simulink model "roll_loop"  (Simulink 9.1)
settings: Solver=VariableStepAuto  StartTime=0.0  StopTime=20  RelTol=1e-3
InitFcn:
  | param_chap6
undefined symbols (not defined in the file): G
libraries: simulink x1, cstblocks x1
settings Model: Creator=leonardopedroso  LastModifiedBy=João Pinto
settings DataIOCC: SaveFormat=Dataset
settings OptimizationCC: LifeSpan=auto
settings DebuggingCC: UnderspecifiedInitializationDetection=Simplified  MergeDetectMultiDrivingBlocksExec=error  SFUnexpectedBacktrackingDiag=error  SFNoUnconditionalDefaultTransitionDiag=error  SFExecutionAtInitializationDiag=warning
settings HardwareCC: ProdBitPerPointer=64  ProdBitPerSizeT=64  ProdBitPerPtrDiffT=64  ProdLargestAtomicFloat=Float  ProdIntDivRoundTo=Zero  ProdEndianess=LittleEndian  ProdWordSize=64  ProdHWDeviceType=Intel->x86-64 (Windows64)
settings ModelReferenceCC: PropagateSignalLabelsOutOfModel=on
settings CodeAppCC: StateflowObjectComments=off
settings GRTTargetCC: TargetLangStandard=C99 (ISO)  CombineOutputUpdateFcns=on  GRTInterface=off
settings ConfigComp: CovMetricSettings=dwe  CovHtmlReporting=off  CovSaveCumulativeToWorkspaceVar=off  CovSaveSingleToWorkspaceVar=off  CovExternalEMLEnable=on

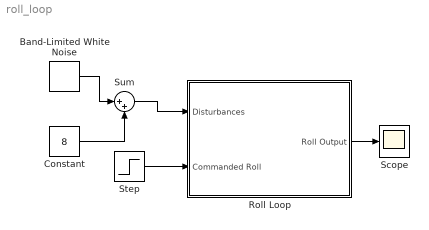
== system roll_loop ==
  Band-Limited White Noise : simulink/Sources/Band-Limited White Noise  Cov=[0.1]  Ts=0.1  seed=[23341]
  Constant : Constant  Value=8
  "Roll Loop " : Subsystem
  Scope : Scope
  Step : Step  After=pi/9  SampleTime=0
  Sum : Sum  Inputs=|++
  wires:
  Step/1 -> "Roll Loop "/2(Commanded Roll)
  "Roll Loop "/1(Roll Output) -> Scope/1
  Band-Limited White Noise/1 -> Sum/1
  Constant/1 -> Sum/2
  Sum/1 -> "Roll Loop "/1("Disturbances ")

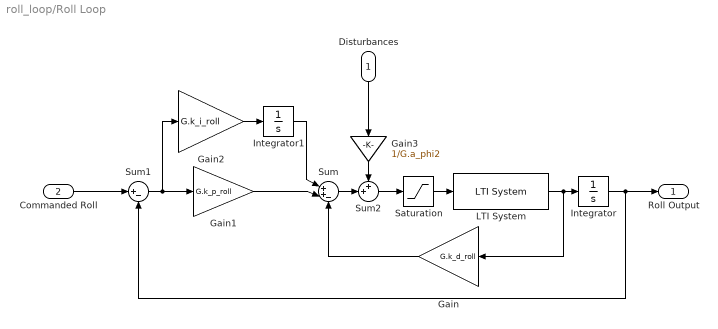
== system roll_loop/Roll Loop  ==
  "Disturbances " : Inport
  Commanded Roll : Inport  Port=2
  Gain : Gain  Gain=G.k_d_roll
  Gain1 : Gain  Gain=G.k_p_roll
  Gain2 : Gain  Gain=G.k_i_roll
  Gain3 : Gain  Gain=1/G.a_phi2
  Integrator : Integrator
  Integrator1 : Integrator
  LTI System : cstblocks/LTI System  sys=T_p_delta_a  IC=[]
  Saturation : Saturate  UpperLimit=G.delta_a_max  LowerLimit=-G.delta_a_max
  Sum : Sum  Inputs=|++-
  Sum1 : Sum  Inputs=|+-
  Sum2 : Sum  Inputs=++|
  Roll Output : Outport
  wires:
  Integrator/1 -> Roll Output/1, Sum1/2
  Gain1/1 -> Sum/2
  Gain/1 -> Sum/3
  Sum1/1 -> Gain2/1, Gain1/1
  Gain2/1 -> Integrator1/1
  Integrator1/1 -> Sum/1
  Commanded Roll/1 -> Sum1/1
  Sum/1 -> Sum2/2
  Gain3/1 -> Sum2/1
  "Disturbances "/1 -> Gain3/1
  Sum2/1 -> Saturation/1
  Saturation/1 -> LTI System/1
  LTI System/1 -> Integrator/1, Gain/1
